simulink model "ImpStepResp"  (R2018b)
settings: Solver=VariableStepAuto  StartTime=0.0  StopTime=120  MaxStep=0.01  RelTol=1e-3
settings Model: Creator=td  LastModifiedBy=td

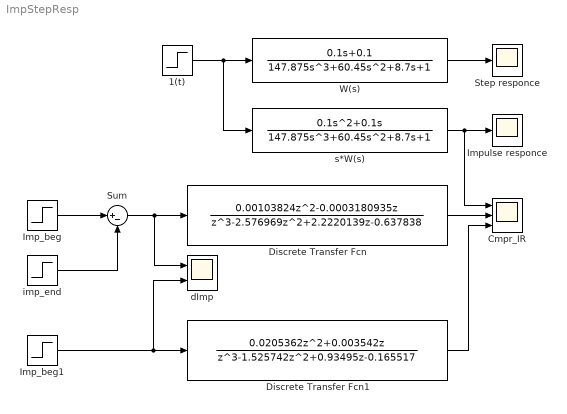
== system ImpStepResp ==
  1(t) : Step  Time=0  SampleTime=0
  Cmpr_IR : Scope  NumInputPorts=3
  Discrete Transfer Fcn : DiscreteTransferFcn  Numerator="[0   0.00103824  -0.0003180935  0]"  Denominator="[1  -2.576969   2.2220139  -0.637838]"  SampleTime=1.1
  Discrete Transfer Fcn1 : DiscreteTransferFcn  Numerator="[0   0.0205362   0.003542   0]"  Denominator="[1  -1.525742   0.93495  -0.165517]"  SampleTime=4.4
  Imp_beg : Step  Time=0  After=1/1.1  SampleTime=0
  Imp_beg1 : Step  Time=4.3  Before=1/4.4  After=0  SampleTime=0
  Impulse responce : Scope
  Step responce : Scope
  Sum : Sum  Inputs=|+-
  W(s) : TransferFcn  Numerator=[0.1 0.1]  Denominator=[147.875 60.45 8.7 1]
  dImp : Scope  NumInputPorts=2
  imp_end : Step  Time=1.1  After=1/1.1  SampleTime=0
  s*W(s) : TransferFcn  Numerator=[0.1 0.1 0]  Denominator=[147.875 60.45 8.7 1]
  wires:
  1(t)/1 -> s*W(s)/1, W(s)/1
  W(s)/1 -> Step responce/1
  s*W(s)/1 -> Cmpr_IR/1, Impulse responce/1
  Discrete Transfer Fcn/1 -> Cmpr_IR/2
  Sum/1 -> dImp/1, Discrete Transfer Fcn/1
  Imp_beg/1 -> Sum/1
  imp_end/1 -> Sum/2
  Imp_beg1/1 -> dImp/2, Discrete Transfer Fcn1/1
  Discrete Transfer Fcn1/1 -> Cmpr_IR/3
